simulink model "BE_synthese_simu1"  (R2018b)
settings: Solver=VariableStepAuto  StartTime=0.0  StopTime=50  RelTol=1e-3
values from neighbouring files (symbols this model uses):
  R = [k -k*a]    [BE3_auto.m]    (also in BE6_7et8_auto.m = 1; BE_synthese.m = [r0 r1 r2])
  S = [1 -1]    [BE3_auto.m]    (also in BE6_7et8_auto.m = 1 / 1 + Gs*Ky_s*Kr_s; BE_synthese.m = [1 (sp1-1) -sp1])
  T = Gs*Ky_s*Kr_s / 1 + Gs*Ky_s*Kr_s    [BE6_7et8_auto.m]    (also in BE_synthese.m = polyval(R,1))
  Te = 0.3    [BE_synthese.m]
settings Model: Creator=piffercg  LastModifiedBy=piffercg

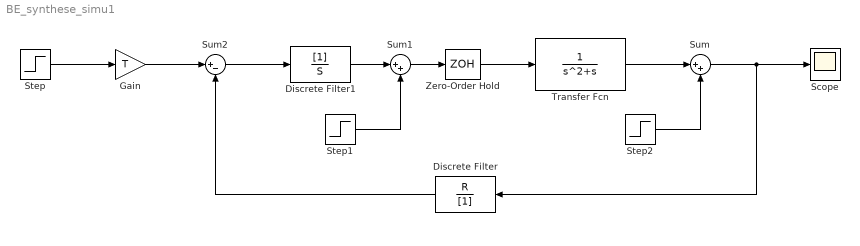
== system BE_synthese_simu1 ==
  Discrete Filter : DiscreteFilter  Numerator=R  Denominator=[1]
  Discrete Filter1 : DiscreteFilter  Denominator=S
  Gain : Gain  Gain=T
  Scope : Scope
  Step : Step  After=5  SampleTime=0
  Step1 : Step  Time=10  After=20  SampleTime=0
  Step2 : Step  Time=30  After=20  SampleTime=0
  Sum : Sum  Inputs=|++
  Sum1 : Sum  Inputs=|++
  Sum2 : Sum  Inputs=|+-
  Transfer Fcn : TransferFcn  Denominator=[1 1 0]
  Zero-Order Hold : ZeroOrderHold  SampleTime=Te
  wires:
  Zero-Order Hold/1 -> Transfer Fcn/1
  Sum/1 -> Discrete Filter/1, Scope/1
  Transfer Fcn/1 -> Sum/1
  Sum1/1 -> Zero-Order Hold/1
  Discrete Filter1/1 -> Sum1/1
  Sum2/1 -> Discrete Filter1/1
  Discrete Filter/1 -> Sum2/2
  Gain/1 -> Sum2/1
  Step/1 -> Gain/1
  Step1/1 -> Sum1/2
  Step2/1 -> Sum/2
